simulink model "MPC_Controller"  (R2025b)
settings: Solver=ode4  StartTime=0.0  StopTime=10  FixedStep=Ts  RelTol=1e-3
undefined symbols (not defined in the file): F_eq, Ts
libraries: uavutilslib x1
settings Model: Creator=david  LastModifiedBy=david

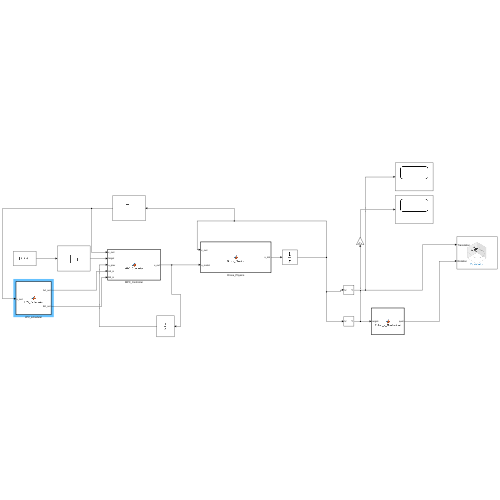
[thumbnail: Simulink's stored preview of the top-level diagram]
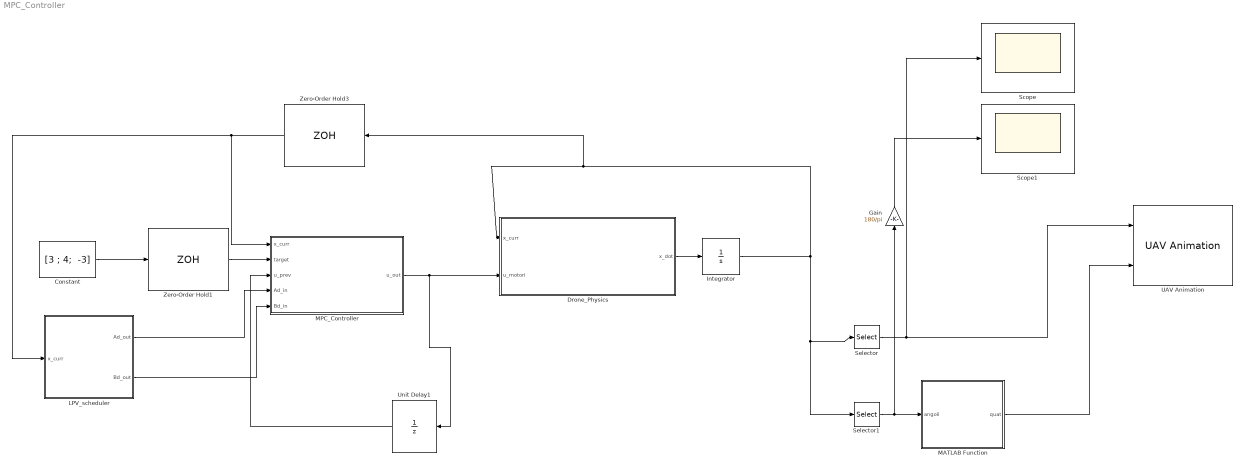
== system MPC_Controller ==
  Constant : Constant  Value="[3 ; 4;  -3]"
  Drone_Physics : MATLAB Function  TreatAsAtomicUnit=on
  Gain : Gain  Gain=180/pi
  Integrator : Integrator  InitialCondition=[0 ; 0 ; 0 ; zeros(9,1)]
  LPV_scheduler : MATLAB Function  TreatAsAtomicUnit=on
  MATLAB Function : MATLAB Function  TreatAsAtomicUnit=on
  MPC_Controller : MATLAB Function  TreatAsAtomicUnit=on
  Scope : Scope
      settings: ActiveDisplayYMinimum=-3.6019198075526266  ActiveDisplayYMaximum=4.1652720045418965
  Scope1 : Scope
      settings: ActiveDisplayYMinimum=-26.887440390939872  ActiveDisplayYMaximum=22.574042876571248
  Selector : Selector  IndexOptions=Index vector (dialog)  Indices=[1 2 3]  OutputSizes=1
  Selector1 : Selector  IndexOptions=Index vector (dialog)  Indices=[4 5 6]  OutputSizes=1
  UAV Animation : uavutilslib/UAV Animation  NumUAV=1  DynamicUAVConfig=off  UAVType=Multirotor  UAVSize=1  UAVColor=[1 0 0]  UAVTrajectoryAlpha=1  InertialZDirection=Down  RotationFormat=Quaternion  DrawMarkers=off  SampleTime=-1
  Unit Delay1 : UnitDelay  InitialCondition=F_eq  SampleTime=Ts  HasFrameUpgradeWarning=on
  Zero-Order Hold1 : ZeroOrderHold  SampleTime=Ts
  Zero-Order Hold3 : ZeroOrderHold  SampleTime=Ts
  wires:
  Drone_Physics/1(x_dot) -> Integrator/1
  MPC_Controller/1(u_out) -> Drone_Physics/2(u_motori), Unit Delay1/1
  Unit Delay1/1 -> MPC_Controller/3(u_prev)
  Selector/1 -> Scope/1, UAV Animation/1
  Selector1/1 -> MATLAB Function/1(angoli), Gain/1
  MATLAB Function/1(quat) -> UAV Animation/2
  Constant/1 -> Zero-Order Hold1/1
  Zero-Order Hold1/1 -> MPC_Controller/2(target)
  Integrator/1 -> Zero-Order Hold3/1, Drone_Physics/1(x_curr), Selector/1, Selector1/1
  Zero-Order Hold3/1 -> LPV_scheduler/1(x_curr), MPC_Controller/1(x_curr)
  Gain/1 -> Scope1/1
  LPV_scheduler/1(Ad_out) -> MPC_Controller/4(Ad_in)
  LPV_scheduler/2(Bd_out) -> MPC_Controller/5(Bd_in)

== matlab function MPC_Controller/Drone_Physics ==
  data: x_curr input; u_motori input; x_dot output
function x_dot = Drone_Physics(x_curr, u_motori)
% Drone_Physics - Dinamica nonlineare del drone per Simulink
% INPUT:
%   x_curr   (12×1) - stato corrente [q; q_dot]
%   u_motori (4×1)  - forze motori [F1,F2,F3,F4] in Newton
% OUTPUT:
%   x_dot    (12×1) - derivata dello stato
%
% Richiede nel workspace: Gamma_num, M_fun, C_fun, B_fun, G_n
% Sample time: CONTINUO (= 0)

    coder.extrinsic('evalin', 'assignin');
    x_dot = zeros(12, 1);

    assignin('base', 'x_sim', double(x_curr(:)));
    assignin('base', 'u_sim', double(u_motori(:)));

    % [T; tau_phi; tau_theta; tau_psi] = Gamma_num * [F1;F2;F3;F4]
    evalin('base', 'U_virt = Gamma_num * u_sim;');

    % Valutazione matrici al punto corrente
    evalin('base', ['Mn = full(M_fun(' ...
        'x_sim(4), x_sim(5), x_sim(6)));']);
    evalin('base', ['Cn = full(C_fun(' ...
        'x_sim(4), x_sim(5), x_sim(6), ' ...
        'x_sim(10), x_sim(11), x_sim(12)));']);
    evalin('base', ['Bn = full(B_fun(' ...
        'x_sim(4), x_sim(5), x_sim(6)));']);

    % Equazione del moto: q_ddot = M^{-1}(-C*q_dot - G + B*U_virt)
    evalin('base', 'q_ddot = Mn \ (-Cn*x_sim(7:12) - G_n + Bn*U_virt);');

    % Derivata dello stato: x_dot = [q_dot; q_ddot]
    evalin('base', 'x_dot_sim = [x_sim(7:12); q_ddot];');

    x_dot = evalin('base', 'double(full(x_dot_sim(:)))');
end

== matlab function MPC_Controller/MPC_Controller ==
  data: x_curr input; u_out output; target input; u_prev input; Ad_in input; Bd_in input
function u_out = MPC_Controller(x_curr, target, u_prev, Ad_in, Bd_in)
% MPC_Controller - Blocco MATLAB Function per Simulink
%
% INPUT:
%   x_curr  (12×1) - stato corrente del drone
%   target  (3×1)  - posizione target [x, y, z]
%   u_prev  (4×1)  - forze motori al passo precedente
%   Ad_in   (12×12)- matrice di stato discretizzata (LPV: può variare)
%   Bd_in   (12×4) - matrice di ingresso discretizzata (LPV: può variare)
%
% OUTPUT:
%   u_out   (4×1)  - forze ottimali per i 4 motori [N]
%
% NOTA: questo blocco richiede che lo script di inizializzazione sia stato
% eseguito prima di avviare Simulink (opti, parametri, F_eq nel workspace)

    % Necessario per usare evalin/assignin in codice generato
    coder.extrinsic('evalin', 'assignin', 'disp', 'fprintf');

    % Inizializzazione output (fallback a hover)
    u_out = zeros(4, 1);

    % ── 1. Passa i dati al workspace base ──────────────────────────────
    assignin('base', 'x_mpc',      double(x_curr(:)));
    assignin('base', 'target_mpc', double(target(:)));
    assignin('base', 'u_prev_mpc', double(u_prev(:)));
    assignin('base', 'Ad_mpc',     double(Ad_in));
    assignin('base', 'Bd_mpc',     double(Bd_in));

    % ── 2. Setta i parametri CasADi ────────────────────────────────────
    % Stato iniziale e target
    evalin('base', 'opti.set_value(x0_param,     x_mpc);');
    evalin('base', 'opti.set_value(target_pos,   target_mpc);');
    evalin('base', 'opti.set_value(u_prev_param, u_prev_mpc);');

    % Matrici dinamica (LPV: aggiornate ad ogni passo)
    evalin('base', 'opti.set_value(Ad_param, Ad_mpc);');
    evalin('base', 'opti.set_value(Bd_param, Bd_mpc);');

    % ── 3. Risolvi il problema MPC ─────────────────────────────────────
    stringa_ottimizzazione = [ ...
        'try;'                                                              ...
        '  sol = opti.solve();'                                             ...
        '  u_opt_val = full(sol.value(U));'                                 ...
        '  u_res = u_opt_val(:, 1);'                                        ...
        '  opti.set_initial(U, [u_opt_val(:,2:end), u_opt_val(:,end)]);'   ... % warm start
        '  mpc_ok = true;'                                                  ...
        'catch e;'                                                          ...
        '  fprintf(''[MPC] IPOPT fallito: %s\n'', e.message);'             ...
        '  u_res = F_eq;'                                                   ... % fallback hover
        '  mpc_ok = false;'                                                 ...
        'end'                                                               ...
    ];
    evalin('base', stringa_ottimizzazione);

    % ── 4. Recupera il risultato ────────────────────────────────────────
    u_out = evalin('base', 'double(u_res(:))');

end

== matlab function MPC_Controller/MATLAB Function ==
  data: angoli input; quat output
function quat = Eulero_a_Quaternioni(angoli)
    % angoli = [phi (roll); theta (pitch); psi (yaw)]
    phi = angoli(1);
    theta = angoli(2);
    psi = angoli(3);
    
    % Formule aerospaziali per il quaternione [qw, qx, qy, qz]
    cy = cos(psi * 0.5);
    sy = sin(psi * 0.5);
    cp = cos(theta * 0.5);
    sp = sin(theta * 0.5);
    cr = cos(phi * 0.5);
    sr = sin(phi * 0.5);
    
    qw = cr * cp * cy + sr * sp * sy;
    qx = sr * cp * cy - cr * sp * sy;
    qy = cr * sp * cy + sr * cp * sy;
    qz = cr * cp * sy - sr * sp * cy;
    
    quat = [qw; qx; qy; qz];
end

== matlab function MPC_Controller/LPV_scheduler ==
  data: x_curr input; Ad_out output; Bd_out output
function [Ad_out, Bd_out] = LPV_Scheduler(x_curr)
% LPV_Scheduler - Aggiorna Ad e Bd in base all'assetto corrente

    coder.extrinsic('evalin', 'assignin');

    Ad_out = zeros(12, 12);
    Bd_out = zeros(12, 4);

    % Passa gli angoli correnti al workspace
    assignin('base', 'phi_lpv',   double(x_curr(4)));
    assignin('base', 'theta_lpv', double(x_curr(5)));
    assignin('base', 'psi_lpv',   double(x_curr(6)));

    % Tutto il calcolo nel workspace base — evita problemi mxArray
    evalin('base', [ ...
        'B_temp = B_lin; '                                                          ...
        'vett_spinta = B_lin(9,:); '                                                ...
        'B_temp(7,:) = vett_spinta*(cos(psi_lpv)*sin(theta_lpv)*cos(phi_lpv) + sin(psi_lpv)*sin(phi_lpv)); ' ...
        'B_temp(8,:) = vett_spinta*(sin(psi_lpv)*sin(theta_lpv)*cos(phi_lpv) - cos(psi_lpv)*sin(phi_lpv)); ' ...
        'B_temp(9,:) = vett_spinta*(cos(theta_lpv)*cos(phi_lpv)); '                 ...
        'sys_k  = ss(A_lin, B_temp, eye(12), zeros(12,4)); '                        ...
        'sys_dk = c2d(sys_k, Ts, ''zoh''); '                                        ...
        'Ad_lpv = sys_dk.A; '                                                       ...
        'Bd_lpv = sys_dk.B; '                                                       ...
    ]);

    Ad_out = evalin('base', 'double(Ad_lpv)');
    Bd_out = evalin('base', 'double(Bd_lpv)');
end
